simulink library "ctrlAllocMatrix3CompCoefSensor_cl"  (R2022a)
settings: Solver=VariableStepAuto  StartTime=0.0  StopTime=10.0  RelTol=1e-3
undefined symbols (not defined in the file or in its folder): fluidDensity, vhcl
libraries: hydroInversionCoefSensor_cl x4
settings Model: Creator=mcobb  LastModifiedBy=adabney
settings SolverCC: AlgebraicLoopSolver=TrustRegion
settings DataIOCC: ReturnWorkspaceOutputs=off
settings DebuggingCC: UnconnectedInputMsg=warning  UnconnectedOutputMsg=warning  UnconnectedLineMsg=warning  SFMachineParentedDataDiag=warning  ArithmeticOperatorsInVariantConditions=warning
settings SFSimCC: CustomCodeUndefinedFunction=UseInterfaceOnly

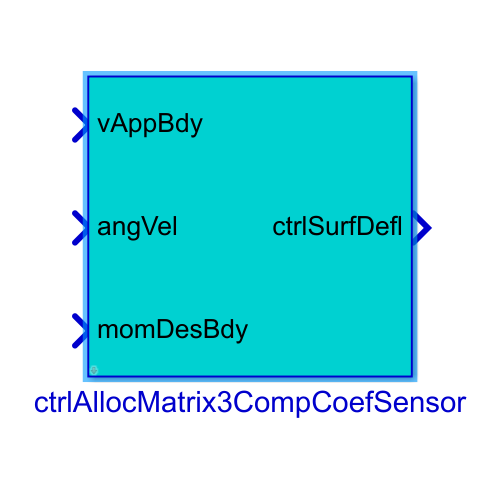
[thumbnail: Simulink's stored preview of the top-level diagram]
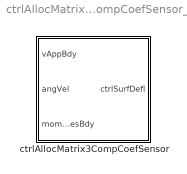
== system ctrlAllocMatrix3CompCoefSensor_cl ==
  ctrlAllocMatrix3CompCoefSensor : Subsystem  mask{aeroStruct=vhcl.struct('OCT.aeroSurf'), fluidDensity=fluidDensity, arms=vhcl.struct('OCT.thrAttch')}
      mask prompts: aeroStruct "Aerodynamic surface structure"; fluidDensity "Fluid density"; arms "Tether Attachment"
      settings: MinAlgLoopOccurrences=on
      mask TypeOptions aeroStruct: momentComponentVector/aeroStruct
      mask TypeOptions fluidDensity: momentComponentVector/fluidDensity

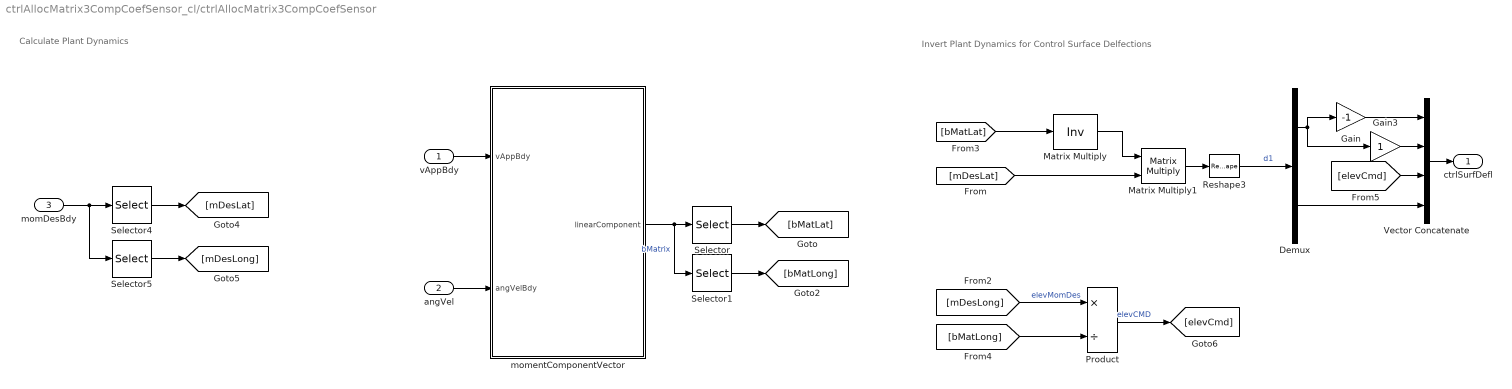
== system ctrlAllocMatrix3CompCoefSensor_cl/ctrlAllocMatrix3CompCoefSensor ==
  note: Invert Plant Dynamics for Control Surface Delfections
  note: Calculate Plant Dynamics
  vAppBdy : Inport
  angVel : Inport  Port=2
  momDesBdy : Inport  Port=3
  Demux : Demux  Outputs=2
  Gain : Gain  Gain=-1
  Gain3 : Gain
  Matrix Multiply : Product  Inputs=/  Multiplication=Matrix(*)
  Matrix Multiply1 : Product  Multiplication=Matrix(*)
  Product : Product  Inputs=*/
  Reshape3 : Reshape
  Selector : Selector  NumberOfDimensions=2  InputPortWidth=3  IndexOptions=Index vector (dialog),Index vector (dialog)  Indices=[1 3],[1 3]  OutputSizes=1,1
  Selector1 : Selector  NumberOfDimensions=2  InputPortWidth=3  IndexOptions=Index vector (dialog),Index vector (dialog)  Indices=2,2  OutputSizes=1,1
  Selector4 : Selector  InputPortWidth=3  IndexOptions=Index vector (dialog)  Indices=[1 3]  OutputSizes=1
  Selector5 : Selector  InputPortWidth=3  IndexOptions=Index vector (dialog)  Indices=2  OutputSizes=1
  Vector Concatenate : Concatenate  NumInputs=4
  momentComponentVector : Subsystem  mask{aeroStruct=aeroStruct, fluidDensity=fluidDensity}
      mask prompts: aeroStruct "Aerodynamic surface structure"; fluidDensity "Fluid density"
      mask help:
      | Input must be an 1×N struct array with fields:
      |     refArea
      |     aeroCentPosVec
      |     spanUnitVec
      |     chordUnitVec
      |     CL
      |     CD
      |     alpha
      |     GainCL
      |     GainCD
      |
      | where N is the number of aerodynamic surfaces
  ctrlSurfDefl : Outport  VectorParamsAs1DForOutWhenUnconnected=off
  wires:
  vAppBdy/1 -> momentComponentVector/1(vAppBdy)
  Gain3/1 -> Vector Concatenate/2
  Vector Concatenate/1 -> ctrlSurfDefl/1
  Demux/1 -> Gain3/1, Gain/1
  Gain/1 -> Vector Concatenate/1
  Reshape3/1 -> Demux/1  "d1"
  angVel/1 -> momentComponentVector/2(angVelBdy)
  [mDesLat] -> Matrix Multiply1/2
  [bMatLat] -> Matrix Multiply/1
  Matrix Multiply1/1 -> Reshape3/1
  momentComponentVector/1(linearComponent) -> Selector1/1, Selector/1  "bMatrix"
  Matrix Multiply/1 -> Matrix Multiply1/1
  Selector/1 -> [bMatLat]
  Selector1/1 -> [bMatLong]
  Selector5/1 -> [mDesLong]
  Selector4/1 -> [mDesLat]
  momDesBdy/1 -> Selector5/1, Selector4/1
  [mDesLong] -> Product/1  "elevMomDes"
  [bMatLong] -> Product/2
  [elevCmd] -> Vector Concatenate/3
  Demux/2 -> Vector Concatenate/4
  Product/1 -> [elevCmd]  "elevCMD"

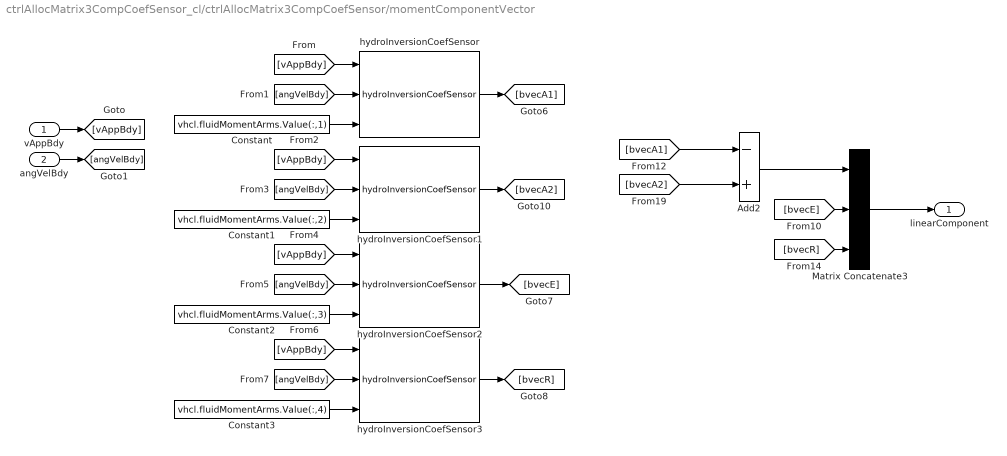
== system ctrlAllocMatrix3CompCoefSensor_cl/ctrlAllocMatrix3CompCoefSensor/momentComponentVector ==
  vAppBdy : Inport
  angVelBdy : Inport  Port=2
  Add2 : Sum  Inputs=-+
  Constant : Constant  Value=vhcl.fluidMomentArms.Value(:,1)
  Constant1 : Constant  Value=vhcl.fluidMomentArms.Value(:,2)
  Constant2 : Constant  Value=vhcl.fluidMomentArms.Value(:,3)
  Constant3 : Constant  Value=vhcl.fluidMomentArms.Value(:,4)
  Matrix Concatenate3 : Concatenate  NumInputs=3  Mode=Multidimensional array  ConcatenateDimension=2
  hydroInversionCoefSensor : hydroInversionCoefSensor_cl/hydroInversionCoefSensor  aeroStruct=vhcl.portWing
  hydroInversionCoefSensor1 : hydroInversionCoefSensor_cl/hydroInversionCoefSensor  aeroStruct=vhcl.stbdWing
  hydroInversionCoefSensor2 : hydroInversionCoefSensor_cl/hydroInversionCoefSensor  aeroStruct=vhcl.hStab
  hydroInversionCoefSensor3 : hydroInversionCoefSensor_cl/hydroInversionCoefSensor  aeroStruct=vhcl.vStab
  linearComponent : Outport
  wires:
  vAppBdy/1 -> [vAppBdy]
  angVelBdy/1 -> [angVelBdy]
  [vAppBdy] -> hydroInversionCoefSensor/1
  [angVelBdy] -> hydroInversionCoefSensor/2
  hydroInversionCoefSensor/1 -> [bvecA1]
  hydroInversionCoefSensor3/1 -> [bvecR]
  hydroInversionCoefSensor1/1 -> [bvecA2]
  [bvecA1] -> Add2/1
  [bvecA2] -> Add2/2
  Constant/1 -> hydroInversionCoefSensor/3
  [bvecR] -> Matrix Concatenate3/3
  Matrix Concatenate3/1 -> linearComponent/1
  Add2/1 -> Matrix Concatenate3/1
  [bvecE] -> Matrix Concatenate3/2
  hydroInversionCoefSensor2/1 -> [bvecE]
  Constant1/1 -> hydroInversionCoefSensor1/3
  [vAppBdy] -> hydroInversionCoefSensor1/1
  [angVelBdy] -> hydroInversionCoefSensor1/2
  Constant2/1 -> hydroInversionCoefSensor2/3
  [vAppBdy] -> hydroInversionCoefSensor2/1
  [angVelBdy] -> hydroInversionCoefSensor2/2
  Constant3/1 -> hydroInversionCoefSensor3/3
  [vAppBdy] -> hydroInversionCoefSensor3/1
  [angVelBdy] -> hydroInversionCoefSensor3/2
